simulink model "DemonstratorSimscape"  (R2020b)
settings: Solver=ode113  StartTime=0.0  StopTime=t_stop*0+20  FixedStep=1e-4
values from neighbouring files (symbols this model uses):
  brkD = 0    [main.m]
  brkI = 1e4    (= 10000)    [main.m]
  brkP = 1e5    (= 100000)    [main.m]
  d_drm = 0.5*d_drum    [main.m]
  d_shm = 0.4*d_sheave    [main.m]
  DeltaCable0 = 0    [main.m]
  Droop_scaling = 0    [main.m]
  eta_sh = 0.015    [main.m]
  filt_NUM = ones(1,200)*0.005    [main.m]
  g = 9.80665    [main.m]
  Iw = 0.5*(W.i + M.in*GB.r^2)    [main.m]
  Kp_mul = 0.3    [main.m]
  Lc0 = abs((T.ph-L.height-P.d-L.z0)*0.001)    [main.m]
  Ls1 = ((T.ph-0.5*W.pd)/1000)    [main.m]
  Ls2 = ((0.5*(T.s2+P.d)-2*P.d)/1000)    [main.m]
  M = 50e3    (= 50000)    [calcGrav.m]
  phi0_drm = -90    [main.m]
  phi0_shm = -90    [main.m]
  r_sheave = P.d*0.5    [main.m]
  s = tf('s')    [calcGrav.m]
  tau_brk = 0.001    [main.m]
  tau_em = 60e-3    (= 0.06)    [calcGrav.m]    (also in main.m)
  tau_m = tau_w/GB.r    [main.m]
  Tmax = 400e3    (= 400000)    [main.m]
  Tn_mul = 10    [main.m]
  x_drm = 0.7*r_drum    [main.m]
  x_shm = 0.7*r_sheave    [main.m]
  z0 = 0    [calcGrav.m]    (also in main.m = L.z0-P.d*0.5-P.d-P.d-L.height-T.h1-T.h2-32)
undefined symbols (not defined in the file or in its folder): C, CA, Controller_sampleTime, DiscIntNeverNeededParam, GB, L, P, Part, T, VFD_acceleration_model_factor, VFD_Adapt_factor_lower_p1458, VFD_Adapt_factor_upper_p1459, VFD_Curr_limit_var_p0641, VFD_Current_limit_p0640, VFD_Id_setp_total_r1624, VFD_Iq, VFD_Kp_n_basic_p1460, VFD_M, VFD_M_accel_T_smooth_p1517, VFD_M_lim_var_fixS_src_p1551, VFD_M_max_lower_p1521, VFD_M_max_lower_scal_p1525, VFD_M_max_up_mot_scal_p1524, VFD_M_max_upper_p1520, VFD_n_act_T_smooth_p1442, VFD_n_ctr_Kp_n_up_scal_p1461, VFD_n_ctr_Tn_n_up_sca_p1463, VFD_n_ctrl_adapt_Kp_lower_p1456, VFD_n_ctrl_adapt_Kp_upper_p1457, VFD_n_ctrl_Adpt_sig_Kp_p1455, VFD_n_ctrl_Kp_scal_p1466, VFD_n_ctrl_n_lower_p1464, VFD_n_ctrl_n_upper_p1465, VFD_n_ctrl_Tn_n_lower_p1462, VFD_n_limit_neg_p1086, VFD_n_limit_pos_p1083, VFD_n_limit_setp_p1063, VFD_n_max_p1082, VFD_n_set_filt_1_T_p1416, VFD_P_max_gen_p1531, VFD_P_max_mot_p1530, VFD_PU_I_outp_max_r0289, VFD_RFG_ramp_down_time_p1121, VFD_RFG_ramp_up_time_p1120, VFD_RFG_t_RD_scal_p1139, VFD_RFG_t_RU_scal_p1138, VSD, W, X, Y, Z
libraries: sm_lib x248, nesl_utility x128, simulink x49, pid_lib x4, cstblocks x2, simulink_extras x2
(part 6 of 10)

== system DemonstratorSimscape/Transmission System/Anchor and Load/FlexDisp_Left/L_23 ==
  L(t)[m] : Inport
  a[m/s^2] : Inport  Port=2
  Constant : Constant  Value=C.EA
  Constant1 : Constant  Value=C.dr
  Constant2 : Constant  Value=Part.m
  Constant3 : Constant  Value=g
  Constant4 : Constant  Value=C.drK
  Gain : Gain  Gain=1/Part.m
  Integrator : Integrator
  Integrator1 : Integrator
  Product : Product  Inputs=*/
  Product{1..3,5} (4 alike) : Product
  Product4 : Product  Inputs=*/
  Product6 : Product  Inputs=/*
  SW_b : ManualSwitch  CurrentSetting=0
  Sqrt : Sqrt  SaturateOnIntegerOverflow=on
  Sum1 : Sum  Inputs=+++
  Sum2 : Sum  Inputs=-+
  F[N] : Outport  VectorParamsAs1DForOutWhenUnconnected=off
  ext [m] : Outport  Port=2  VectorParamsAs1DForOutWhenUnconnected=off
  ext speed [m/s] : Outport  Port=3  VectorParamsAs1DForOutWhenUnconnected=off
  wires:
  L(t)[m]/1 -> Product/2
  Constant/1 -> Product/1
  Product2/1 -> Sum1/1
  Product3/1 -> Sum1/3
  Sum2/1 -> Product4/1, F[N]/1
  Product/1 -> Gain/1, Product2/2  "k"
  Constant2/1 -> Product4/2, Product5/2, Product3/2
  Integrator/1 -> ext speed [m/s]/1, Product1/2, Integrator1/1
  Integrator1/1 -> Product2/1, ext [m]/1
  Product4/1 -> Integrator/1
  Product1/1 -> Sum1/2
  a[m/s^2]/1 -> Product3/1
  Sum1/1 -> Sum2/1
  Product5/1 -> Sum2/2
  Constant3/1 -> Product5/1
  Gain/1 -> Sqrt/1
  Sqrt/1 -> Product6/1
  Constant4/1 -> Product6/2
  Constant1/1 -> SW_b/2
  Product6/1 -> SW_b/1
  SW_b/1 -> Product1/1

== system DemonstratorSimscape/Transmission System/Anchor and Load/FlexDisp_Left/L_34 ==
  L(t)[m] : Inport
  a[m/s^2] : Inport  Port=2
  Constant : Constant  Value=C.EA
  Constant1 : Constant  Value=C.dr
  Constant2 : Constant  Value=Part.m
  Constant3 : Constant  Value=g
  Constant4 : Constant  Value=C.drK
  Gain : Gain  Gain=1/Part.m
  Integrator : Integrator
  Integrator1 : Integrator
  Product : Product  Inputs=*/
  Product{1..3,5} (4 alike) : Product
  Product4 : Product  Inputs=*/
  Product6 : Product  Inputs=/*
  SW_b : ManualSwitch  CurrentSetting=0
  Sqrt : Sqrt  SaturateOnIntegerOverflow=on
  Sum1 : Sum  Inputs=+++
  Sum2 : Sum  Inputs=-+
  F[N] : Outport  VectorParamsAs1DForOutWhenUnconnected=off
  ext [m] : Outport  Port=2  VectorParamsAs1DForOutWhenUnconnected=off
  ext speed [m/s] : Outport  Port=3  VectorParamsAs1DForOutWhenUnconnected=off
  wires:
  L(t)[m]/1 -> Product/2
  Constant/1 -> Product/1
  Product2/1 -> Sum1/1
  Product3/1 -> Sum1/3
  Sum2/1 -> Product4/1, F[N]/1
  Product/1 -> Gain/1, Product2/2  "k"
  Constant2/1 -> Product4/2, Product5/2, Product3/2
  Integrator/1 -> ext speed [m/s]/1, Product1/2, Integrator1/1
  Integrator1/1 -> Product2/1, ext [m]/1
  Product4/1 -> Integrator/1
  Product1/1 -> Sum1/2
  a[m/s^2]/1 -> Product3/1
  Sum1/1 -> Sum2/1
  Product5/1 -> Sum2/2
  Constant3/1 -> Product5/1
  Gain/1 -> Sqrt/1
  Sqrt/1 -> Product6/1
  Constant4/1 -> Product6/2
  Constant1/1 -> SW_b/2
  Product6/1 -> SW_b/1
  SW_b/1 -> Product1/1

== system DemonstratorSimscape/Transmission System/Anchor and Load/FlexDisp_Left/L_w1 ==
  L(t)[m] : Inport
  a[m/s^2] : Inport  Port=2
  Constant : Constant  Value=C.EA
  Constant1 : Constant  Value=C.dr
  Constant2 : Constant  Value=Part.m
  Constant3 : Constant  Value=g
  Constant4 : Constant  Value=C.drK
  Gain : Gain  Gain=1/Part.m
  Integrator : Integrator
  Integrator1 : Integrator
  Product : Product  Inputs=*/
  Product{1..3,5} (4 alike) : Product
  Product4 : Product  Inputs=*/
  Product6 : Product  Inputs=/*
  SW_b : ManualSwitch  CurrentSetting=0
  Sqrt : Sqrt  SaturateOnIntegerOverflow=on
  Sum1 : Sum  Inputs=+++
  Sum2 : Sum  Inputs=-+
  F[N] : Outport  VectorParamsAs1DForOutWhenUnconnected=off
  ext [m] : Outport  Port=2  VectorParamsAs1DForOutWhenUnconnected=off
  ext speed [m/s] : Outport  Port=3  VectorParamsAs1DForOutWhenUnconnected=off
  wires:
  L(t)[m]/1 -> Product/2
  Constant/1 -> Product/1
  Product2/1 -> Sum1/1
  Product3/1 -> Sum1/3
  Sum2/1 -> Product4/1, F[N]/1
  Product/1 -> Gain/1, Product2/2  "k"
  Constant2/1 -> Product4/2, Product5/2, Product3/2
  Integrator/1 -> ext speed [m/s]/1, Product1/2, Integrator1/1
  Integrator1/1 -> Product2/1, ext [m]/1
  Product4/1 -> Integrator/1
  Product1/1 -> Sum1/2
  a[m/s^2]/1 -> Product3/1
  Sum1/1 -> Sum2/1
  Product5/1 -> Sum2/2
  Constant3/1 -> Product5/1
  Gain/1 -> Sqrt/1
  Sqrt/1 -> Product6/1
  Constant4/1 -> Product6/2
  Constant1/1 -> SW_b/2
  Product6/1 -> SW_b/1
  SW_b/1 -> Product1/1

== system DemonstratorSimscape/Transmission System/Anchor and Load/FlexDisp_Right/L_54 ==
  L(t)[m] : Inport
  a[m/s^2] : Inport  Port=2
  Constant : Constant  Value=C.EA
  Constant1 : Constant  Value=C.dr
  Constant2 : Constant  Value=Part.m
  Constant3 : Constant  Value=g
  Constant4 : Constant  Value=C.drK
  Gain : Gain  Gain=1/Part.m
  Integrator : Integrator
  Integrator1 : Integrator
  Product : Product  Inputs=*/
  Product{1..3,5} (4 alike) : Product
  Product4 : Product  Inputs=*/
  Product6 : Product  Inputs=/*
  SW_b : ManualSwitch  CurrentSetting=0
  Sqrt : Sqrt  SaturateOnIntegerOverflow=on
  Sum1 : Sum  Inputs=+++
  Sum2 : Sum  Inputs=-+
  F[N] : Outport  VectorParamsAs1DForOutWhenUnconnected=off
  ext [m] : Outport  Port=2  VectorParamsAs1DForOutWhenUnconnected=off
  ext speed [m/s] : Outport  Port=3  VectorParamsAs1DForOutWhenUnconnected=off
  wires:
  L(t)[m]/1 -> Product/2
  Constant/1 -> Product/1
  Product2/1 -> Sum1/1
  Product3/1 -> Sum1/3
  Sum2/1 -> Product4/1, F[N]/1
  Product/1 -> Gain/1, Product2/2  "k"
  Constant2/1 -> Product4/2, Product5/2, Product3/2
  Integrator/1 -> ext speed [m/s]/1, Product1/2, Integrator1/1
  Integrator1/1 -> Product2/1, ext [m]/1
  Product4/1 -> Integrator/1
  Product1/1 -> Sum1/2
  a[m/s^2]/1 -> Product3/1
  Sum1/1 -> Sum2/1
  Product5/1 -> Sum2/2
  Constant3/1 -> Product5/1
  Gain/1 -> Sqrt/1
  Sqrt/1 -> Product6/1
  Constant4/1 -> Product6/2
  Constant1/1 -> SW_b/2
  Product6/1 -> SW_b/1
  SW_b/1 -> Product1/1

== system DemonstratorSimscape/Transmission System/Anchor and Load/FlexDisp_Right/L_65 ==
  L(t)[m] : Inport
  a[m/s^2] : Inport  Port=2
  Constant : Constant  Value=C.EA
  Constant1 : Constant  Value=C.dr
  Constant2 : Constant  Value=Part.m
  Constant3 : Constant  Value=g
  Constant4 : Constant  Value=C.drK
  Gain : Gain  Gain=1/Part.m
  Integrator : Integrator
  Integrator1 : Integrator
  Product : Product  Inputs=*/
  Product{1..3,5} (4 alike) : Product
  Product4 : Product  Inputs=*/
  Product6 : Product  Inputs=/*
  SW_b : ManualSwitch  CurrentSetting=0
  Sqrt : Sqrt  SaturateOnIntegerOverflow=on
  Sum1 : Sum  Inputs=+++
  Sum2 : Sum  Inputs=-+
  F[N] : Outport  VectorParamsAs1DForOutWhenUnconnected=off
  ext [m] : Outport  Port=2  VectorParamsAs1DForOutWhenUnconnected=off
  ext speed [m/s] : Outport  Port=3  VectorParamsAs1DForOutWhenUnconnected=off
  wires:
  L(t)[m]/1 -> Product/2
  Constant/1 -> Product/1
  Product2/1 -> Sum1/1
  Product3/1 -> Sum1/3
  Sum2/1 -> Product4/1, F[N]/1
  Product/1 -> Gain/1, Product2/2  "k"
  Constant2/1 -> Product4/2, Product5/2, Product3/2
  Integrator/1 -> ext speed [m/s]/1, Product1/2, Integrator1/1
  Integrator1/1 -> Product2/1, ext [m]/1
  Product4/1 -> Integrator/1
  Product1/1 -> Sum1/2
  a[m/s^2]/1 -> Product3/1
  Sum1/1 -> Sum2/1
  Product5/1 -> Sum2/2
  Constant3/1 -> Product5/1
  Gain/1 -> Sqrt/1
  Sqrt/1 -> Product6/1
  Constant4/1 -> Product6/2
  Constant1/1 -> SW_b/2
  Product6/1 -> SW_b/1
  SW_b/1 -> Product1/1

== system DemonstratorSimscape/Transmission System/Anchor and Load/FlexDisp_Right/L_76 ==
  L(t)[m] : Inport
  a[m/s^2] : Inport  Port=2
  Constant : Constant  Value=C.EA
  Constant1 : Constant  Value=C.dr
  Constant2 : Constant  Value=Part.m
  Constant3 : Constant  Value=g
  Constant4 : Constant  Value=C.drK
  Gain : Gain  Gain=1/Part.m
  Integrator : Integrator
  Integrator1 : Integrator
  Product : Product  Inputs=*/
  Product{1..3,5} (4 alike) : Product
  Product4 : Product  Inputs=*/
  Product6 : Product  Inputs=/*
  SW_b : ManualSwitch  CurrentSetting=0
  Sqrt : Sqrt  SaturateOnIntegerOverflow=on
  Sum1 : Sum  Inputs=+++
  Sum2 : Sum  Inputs=-+
  F[N] : Outport  VectorParamsAs1DForOutWhenUnconnected=off
  ext [m] : Outport  Port=2  VectorParamsAs1DForOutWhenUnconnected=off
  ext speed [m/s] : Outport  Port=3  VectorParamsAs1DForOutWhenUnconnected=off
  wires:
  L(t)[m]/1 -> Product/2
  Constant/1 -> Product/1
  Product2/1 -> Sum1/1
  Product3/1 -> Sum1/3
  Sum2/1 -> Product4/1, F[N]/1
  Product/1 -> Gain/1, Product2/2  "k"
  Constant2/1 -> Product4/2, Product5/2, Product3/2
  Integrator/1 -> ext speed [m/s]/1, Product1/2, Integrator1/1
  Integrator1/1 -> Product2/1, ext [m]/1
  Product4/1 -> Integrator/1
  Product1/1 -> Sum1/2
  a[m/s^2]/1 -> Product3/1
  Sum1/1 -> Sum2/1
  Product5/1 -> Sum2/2
  Constant3/1 -> Product5/1
  Gain/1 -> Sqrt/1
  Sqrt/1 -> Product6/1
  Constant4/1 -> Product6/2
  Constant1/1 -> SW_b/2
  Product6/1 -> SW_b/1
  SW_b/1 -> Product1/1

== system DemonstratorSimscape/Transmission System/Anchor and Load/FlexDisp_Right/L_w7 ==
  L(t)[m] : Inport
  a[m/s^2] : Inport  Port=2
  Constant : Constant  Value=C.EA
  Constant1 : Constant  Value=C.dr
  Constant2 : Constant  Value=Part.m
  Constant3 : Constant  Value=g
  Constant4 : Constant  Value=C.drK
  Gain : Gain  Gain=1/Part.m
  Integrator : Integrator
  Integrator1 : Integrator
  Product : Product  Inputs=*/
  Product{1..3,5} (4 alike) : Product
  Product4 : Product  Inputs=*/
  Product6 : Product  Inputs=/*
  SW_b : ManualSwitch  CurrentSetting=0
  Sqrt : Sqrt  SaturateOnIntegerOverflow=on
  Sum1 : Sum  Inputs=+++
  Sum2 : Sum  Inputs=-+
  F[N] : Outport  VectorParamsAs1DForOutWhenUnconnected=off
  ext [m] : Outport  Port=2  VectorParamsAs1DForOutWhenUnconnected=off
  ext speed [m/s] : Outport  Port=3  VectorParamsAs1DForOutWhenUnconnected=off
  wires:
  L(t)[m]/1 -> Product/2
  Constant/1 -> Product/1
  Product2/1 -> Sum1/1
  Product3/1 -> Sum1/3
  Sum2/1 -> Product4/1, F[N]/1
  Product/1 -> Gain/1, Product2/2  "k"
  Constant2/1 -> Product4/2, Product5/2, Product3/2
  Integrator/1 -> ext speed [m/s]/1, Product1/2, Integrator1/1
  Integrator1/1 -> Product2/1, ext [m]/1
  Product4/1 -> Integrator/1
  Product1/1 -> Sum1/2
  a[m/s^2]/1 -> Product3/1
  Sum1/1 -> Sum2/1
  Product5/1 -> Sum2/2
  Constant3/1 -> Product5/1
  Gain/1 -> Sqrt/1
  Sqrt/1 -> Product6/1
  Constant4/1 -> Product6/2
  Constant1/1 -> SW_b/2
  Product6/1 -> SW_b/1
  SW_b/1 -> Product1/1

== system DemonstratorSimscape/Transmission System/Anchor and Load/Load/DOUBLE ==
  cable mass : Inport
  " 1" : sm_lib/Frames and Transforms/Rigid Transform  TranslationMethod=Cartesian  TranslationStandardOffset=0  TranslationLengthUnit=mm  TranslationStandardAxis=+Z  TranslationCartesianOffset=[0 -P.d*0.5 0 ]  TranslationROffset=0  TranslationROffsetUnits=m  TranslationZOffset=0  TranslationZOffsetUnits=m  TranslationThetaOffset=0  TranslationThetaOffsetUnits=deg  RotationMethod=None  RotationAngleUnits=deg  RotationStandardAxis=+Z  RotationAngle=0  RotationArbitraryAxis=[0 0 1]  FollAlignAxisA=+X  BaseAlignAxisA=+Y  FollAlignAxisB=+Y  BaseAlignAxisB=+Z  RotationSequenceAxes=FollowerAxes  RotationSequence=XYX  RotationSequenceAngles=[0 0 0]  RotationSequenceAnglesUnits=deg  RotationMatrix=[1 0 0; 0 1 0; 0 0 1]
  " 2" : sm_lib/Frames and Transforms/Rigid Transform  TranslationMethod=Cartesian  TranslationStandardOffset=0  TranslationLengthUnit=mm  TranslationStandardAxis=+Z  TranslationCartesianOffset=[0 -P.d*0.5 0 ]  TranslationROffset=0  TranslationROffsetUnits=m  TranslationZOffset=0  TranslationZOffsetUnits=m  TranslationThetaOffset=0  TranslationThetaOffsetUnits=deg  RotationMethod=None  RotationAngleUnits=deg  RotationStandardAxis=+Z  RotationAngle=0  RotationArbitraryAxis=[0 0 1]  FollAlignAxisA=+X  BaseAlignAxisA=+Y  FollAlignAxisB=+Y  BaseAlignAxisB=+Z  RotationSequenceAxes=FollowerAxes  RotationSequence=XYX  RotationSequenceAngles=[0 0 0]  RotationSequenceAnglesUnits=deg  RotationMatrix=[1 0 0; 0 1 0; 0 0 1]
  Cable_Left : Subsystem
  Cable_Right : Subsystem
  Half-Place R : sm_lib/Body Elements/Brick Solid  GraphicAmbientColor=[0.15 0.15 0.15 1.0]  BasedOnType=Mass  BrickDimensions=[L.ap*2 P.d 1.5*P.h]  BrickDimensionUnits=mm  CenterOfMass=[0 0 0]  CenterOfMassUnits=m  GraphicDiffuseColor=c.plate  Density=0  DensityUnits=g/cm^3  DoExposeReferenceFrame=on  GraphicEmissiveColor=[0.0 0.0 0.0 1.0]  ExportEntireGeometry=off  SerializedFrames=<Frames/>  MarkerShape=Sphere  MarkerSize=10  GraphicType=FromGeometry  InertiaType=CalculateFromGeometry  Mass=L.cpmass/2  MassUnits=kg  MomentsOfInertia=[1 1 1]  MomentsOfInertiaUnits=kg*m^2  GraphicOpacity=c.opac  ProductsOfInertia=[0 0 0]  ProductsOfInertiaUnits=kg*m^2  GraphicShininess=75  GraphicSpecularColor=[0.5 0.5 0.5 1.0]  GraphicVisPropType=SimpleVisualProperties
  Half-Plate L : sm_lib/Body Elements/Brick Solid  GraphicAmbientColor=[0.15 0.15 0.15 1.0]  BasedOnType=Mass  BrickDimensions=[L.ap*2 P.d 1.5*P.h]  BrickDimensionUnits=mm  CenterOfMass=[0 0 0]  CenterOfMassUnits=m  GraphicDiffuseColor=c.plate  Density=0  DensityUnits=g/cm^3  DoExposeReferenceFrame=on  GraphicEmissiveColor=[0.0 0.0 0.0 1.0]  ExportEntireGeometry=off  SerializedFrames=<Frames/>  MarkerShape=Sphere  MarkerSize=10  GraphicType=FromGeometry  InertiaType=CalculateFromGeometry  Mass=L.cpmass/2  MassUnits=kg  MomentsOfInertia=[1 1 1]  MomentsOfInertiaUnits=kg*m^2  GraphicOpacity=c.opac  ProductsOfInertia=[0 0 0]  ProductsOfInertiaUnits=kg*m^2  GraphicShininess=75  GraphicSpecularColor=[0.5 0.5 0.5 1.0]  GraphicVisPropType=SimpleVisualProperties
  Load blue : sm_lib/Body Elements/Brick Solid  GraphicAmbientColor=[0.15 0.15 0.15 1.0]  BasedOnType=Mass  BrickDimensions="[L.width L.height  L.depth]"  BrickDimensionUnits=mm  CenterOfMass=[0 0 0]  CenterOfMassUnits=m  GraphicDiffuseColor=c.Rload  Density=L.den  DensityUnits=g/cm^3  DoExposeReferenceFrame=off  GraphicEmissiveColor=[0.0 0.0 0.0 1.0]  ExportEntireGeometry=off  SerializedFrames=<Frames><Frame><Id>Frame1</Id><Value><Name>F</Name><Origin><Source>ReferenceFrame</Source><FeatureName></FeatureName></Origin><PrimaryAxis><DefinedDirection>+Z</DefinedDirection><Source>ReferenceFrame</Source><SourceDirection>+Z</SourceDirection><FeatureName></FeatureName></PrimaryAxis><SecondaryAxis><DefinedDirection>+X</DefinedDirection><Source>ReferenceFrame</Source><SourceDirection>+X</SourceDirection><FeatureName></FeatureName></SecondaryAxis></Value></Frame></Frames>  MarkerShape=Sphere  MarkerSize=10  GraphicType=FromGeometry  InertiaType=CalculateFromGeometry  Mass=L.mass  MassUnits=kg  MomentsOfInertia=[0 0 0]  MomentsOfInertiaUnits=kg*m^2  GraphicOpacity=1.0  ProductsOfInertia=[0 0 0]  ProductsOfInertiaUnits=kg*m^2  GraphicShininess=75  GraphicSpecularColor=[0.5 0.5 0.5 1.0]  GraphicVisPropType=SimpleVisualProperties
  Load init position1 : sm_lib/Frames and Transforms/Rigid Transform  TranslationMethod=Cartesian  TranslationStandardOffset=0  TranslationLengthUnit=mm  TranslationStandardAxis=+Z  TranslationCartesianOffset=[0 -P.d*0.5-L.height*0.5 -P.h*.5 ]  TranslationROffset=0  TranslationROffsetUnits=m  TranslationZOffset=0  TranslationZOffsetUnits=m  TranslationThetaOffset=0  TranslationThetaOffsetUnits=deg  RotationMethod=StandardAxis  RotationAngleUnits=deg  RotationStandardAxis=+Y  RotationAngle=180  RotationArbitraryAxis=[0 0 1]  FollAlignAxisA=+X  BaseAlignAxisA=+Y  FollAlignAxisB=+Y  BaseAlignAxisB=+Z  RotationSequenceAxes=FollowerAxes  RotationSequence=XYX  RotationSequenceAngles=[0 0 0]  RotationSequenceAnglesUnits=deg  RotationMatrix=[1 0 0; 0 1 0; 0 0 1]
  Load init position2 : sm_lib/Frames and Transforms/Rigid Transform  TranslationMethod=Cartesian  TranslationStandardOffset=0  TranslationLengthUnit=mm  TranslationStandardAxis=+Z  TranslationCartesianOffset=[0 -L.height*.5-P.d 0 ]  TranslationROffset=0  TranslationROffsetUnits=m  TranslationZOffset=0  TranslationZOffsetUnits=m  TranslationThetaOffset=0  TranslationThetaOffsetUnits=deg  RotationMethod=None  RotationAngleUnits=deg  RotationStandardAxis=+X  RotationAngle=180  RotationArbitraryAxis=[0 0 1]  FollAlignAxisA=+X  BaseAlignAxisA=+Y  FollAlignAxisB=+Y  BaseAlignAxisB=+Z  RotationSequenceAxes=FollowerAxes  RotationSequence=XYX  RotationSequenceAngles=[0 0 0]  RotationSequenceAnglesUnits=deg  RotationMatrix=[1 0 0; 0 1 0; 0 0 1]
  Load init position3 : sm_lib/Frames and Transforms/Rigid Transform  TranslationMethod=Cartesian  TranslationStandardOffset=0  TranslationLengthUnit=mm  TranslationStandardAxis=+Z  TranslationCartesianOffset=[0 -L.height*.5-P.d 0 ]  TranslationROffset=0  TranslationROffsetUnits=m  TranslationZOffset=0  TranslationZOffsetUnits=m  TranslationThetaOffset=0  TranslationThetaOffsetUnits=deg  RotationMethod=None  RotationAngleUnits=deg  RotationStandardAxis=+X  RotationAngle=180  RotationArbitraryAxis=[0 0 1]  FollAlignAxisA=+X  BaseAlignAxisA=+Y  FollAlignAxisB=+Y  BaseAlignAxisB=+Z  RotationSequenceAxes=FollowerAxes  RotationSequence=XYX  RotationSequenceAngles=[0 0 0]  RotationSequenceAnglesUnits=deg  RotationMatrix=[1 0 0; 0 1 0; 0 0 1]
  Load init position4 : sm_lib/Frames and Transforms/Rigid Transform  TranslationMethod=Cartesian  TranslationStandardOffset=0  TranslationLengthUnit=mm  TranslationStandardAxis=+Z  TranslationCartesianOffset=[0 -P.d*0.5-L.height*0.5 -P.h*.5 ]  TranslationROffset=0  TranslationROffsetUnits=m  TranslationZOffset=0  TranslationZOffsetUnits=m  TranslationThetaOffset=0  TranslationThetaOffsetUnits=deg  RotationMethod=StandardAxis  RotationAngleUnits=deg  RotationStandardAxis=+Y  RotationAngle=180  RotationArbitraryAxis=[0 0 1]  FollAlignAxisA=+X  BaseAlignAxisA=+Y  FollAlignAxisB=+Y  BaseAlignAxisB=+Z  RotationSequenceAxes=FollowerAxes  RotationSequence=XYX  RotationSequenceAngles=[0 0 0]  RotationSequenceAnglesUnits=deg  RotationMatrix=[1 0 0; 0 1 0; 0 0 1]
  Load yellow : sm_lib/Body Elements/Brick Solid  GraphicAmbientColor=[0.15 0.15 0.15 1.0]  BasedOnType=Mass  BrickDimensions="[L.width L.height  L.depth]"  BrickDimensionUnits=mm  CenterOfMass=[0 0 0]  CenterOfMassUnits=m  GraphicDiffuseColor=[1.0 1.0 0.0]  Density=L.den  DensityUnits=g/cm^3  DoExposeReferenceFrame=off  GraphicEmissiveColor=[0.0 0.0 0.0 1.0]  ExportEntireGeometry=off  SerializedFrames=<Frames><Frame><Id>Frame1</Id><Value><Name>F</Name><Origin><Source>ReferenceFrame</Source><FeatureName></FeatureName></Origin><PrimaryAxis><DefinedDirection>+Z</DefinedDirection><Source>ReferenceFrame</Source><SourceDirection>+Z</SourceDirection><FeatureName></FeatureName></PrimaryAxis><SecondaryAxis><DefinedDirection>+X</DefinedDirection><Source>ReferenceFrame</Source><SourceDirection>+X</SourceDirection><FeatureName></FeatureName></SecondaryAxis></Value></Frame></Frames>  MarkerShape=Sphere  MarkerSize=10  GraphicType=FromGeometry  InertiaType=CalculateFromGeometry  Mass=L.mass  MassUnits=kg  MomentsOfInertia=[0 0 0]  MomentsOfInertiaUnits=kg*m^2  GraphicOpacity=1.0  ProductsOfInertia=[0 0 0]  ProductsOfInertiaUnits=kg*m^2  GraphicShininess=75  GraphicSpecularColor=[0.5 0.5 0.5 1.0]  GraphicVisPropType=SimpleVisualProperties
  Load1 Rotation1 : sm_lib/Frames and Transforms/Rigid Transform  TranslationMethod=None  TranslationStandardOffset=0  TranslationLengthUnit=m  TranslationStandardAxis=+Z  TranslationCartesianOffset=[0 0 0]  TranslationROffset=0  TranslationROffsetUnits=m  TranslationZOffset=0  TranslationZOffsetUnits=m  TranslationThetaOffset=0  TranslationThetaOffsetUnits=deg  RotationMethod=StandardAxis  RotationAngleUnits=deg  RotationStandardAxis=+X  RotationAngle=90  RotationArbitraryAxis=[0 0 1]  FollAlignAxisA=+Y  BaseAlignAxisA=-Z  FollAlignAxisB=+X  BaseAlignAxisB=+X  RotationSequenceAxes=FollowerAxes  RotationSequence=XYX  RotationSequenceAngles=[0 0 0]  RotationSequenceAnglesUnits=deg  RotationMatrix=[1 0 0; 0 1 0; 0 0 1]
  Load1 Rotation2 : sm_lib/Frames and Transforms/Rigid Transform  TranslationMethod=None  TranslationStandardOffset=0  TranslationLengthUnit=m  TranslationStandardAxis=+Z  TranslationCartesianOffset=[0 0 0]  TranslationROffset=0  TranslationROffsetUnits=m  TranslationZOffset=0  TranslationZOffsetUnits=m  TranslationThetaOffset=0  TranslationThetaOffsetUnits=deg  RotationMethod=StandardAxis  RotationAngleUnits=deg  RotationStandardAxis=+X  RotationAngle=90  RotationArbitraryAxis=[0 0 1]  FollAlignAxisA=+Y  BaseAlignAxisA=-Z  FollAlignAxisB=+X  BaseAlignAxisB=+X  RotationSequenceAxes=FollowerAxes  RotationSequence=XYX  RotationSequenceAngles=[0 0 0]  RotationSequenceAnglesUnits=deg  RotationMatrix=[1 0 0; 0 1 0; 0 0 1]
  Planar Load1 : Subsystem
  Planar Load2 : Subsystem
  Rigid Transform1 : sm_lib/Frames and Transforms/Rigid Transform  TranslationMethod=Cartesian  TranslationStandardOffset=0  TranslationLengthUnit=mm  TranslationStandardAxis=+Z  TranslationCartesianOffset=[0 0.5*T.rs 0]  TranslationROffset=0  TranslationROffsetUnits=m  TranslationZOffset=0  TranslationZOffsetUnits=m  TranslationThetaOffset=0  TranslationThetaOffsetUnits=deg  RotationMethod=StandardAxis  RotationAngleUnits=deg  RotationStandardAxis=+Y  RotationAngle=180  RotationArbitraryAxis=[1 0 0]  FollAlignAxisA=+X  BaseAlignAxisA=+Y  FollAlignAxisB=+Y  BaseAlignAxisB=+Z  RotationSequenceAxes=FollowerAxes  RotationSequence=XYX  RotationSequenceAngles=[0 0 0]  RotationSequenceAnglesUnits=deg  RotationMatrix=[1 0 0; 0 1 0; 0 0 1]
  Rigid Transform2 : sm_lib/Frames and Transforms/Rigid Transform  TranslationMethod=Cartesian  TranslationStandardOffset=0  TranslationLengthUnit=mm  TranslationStandardAxis=+Z  TranslationCartesianOffset=[0 0.5*T.rs 0]  TranslationROffset=0  TranslationROffsetUnits=m  TranslationZOffset=0  TranslationZOffsetUnits=m  TranslationThetaOffset=0  TranslationThetaOffsetUnits=deg  RotationMethod=StandardAxis  RotationAngleUnits=deg  RotationStandardAxis=+Y  RotationAngle=180  RotationArbitraryAxis=[1 0 0]  FollAlignAxisA=+X  BaseAlignAxisA=+Y  FollAlignAxisB=+Y  BaseAlignAxisB=+Z  RotationSequenceAxes=FollowerAxes  RotationSequence=XYX  RotationSequenceAngles=[0 0 0]  RotationSequenceAnglesUnits=deg  RotationMatrix=[1 0 0; 0 1 0; 0 0 1]
  Rigid Transform3 : sm_lib/Frames and Transforms/Rigid Transform  TranslationMethod=Cartesian  TranslationStandardOffset=0  TranslationLengthUnit=mm  TranslationStandardAxis=+Z  TranslationCartesianOffset=[-0.5*(P.Bd+P.d) 0 0]  TranslationROffset=0  TranslationROffsetUnits=m  TranslationZOffset=0  TranslationZOffsetUnits=m  TranslationThetaOffset=0  TranslationThetaOffsetUnits=deg  RotationMethod=StandardAxis  RotationAngleUnits=deg  RotationStandardAxis=+Z  RotationAngle=180  RotationArbitraryAxis=[1 0 0]  FollAlignAxisA=+X  BaseAlignAxisA=+Y  FollAlignAxisB=+Y  BaseAlignAxisB=+Z  RotationSequenceAxes=FollowerAxes  RotationSequence=XYX  RotationSequenceAngles=[0 0 0]  RotationSequenceAnglesUnits=deg  RotationMatrix=[1 0 0; 0 1 0; 0 0 1]
  Rigid Transform4 : sm_lib/Frames and Transforms/Rigid Transform  TranslationMethod=Cartesian  TranslationStandardOffset=0  TranslationLengthUnit=mm  TranslationStandardAxis=+Z  TranslationCartesianOffset=[0.5*(P.Bd+P.d) 0 0]  TranslationROffset=0  TranslationROffsetUnits=m  TranslationZOffset=0  TranslationZOffsetUnits=m  TranslationThetaOffset=0  TranslationThetaOffsetUnits=deg  RotationMethod=StandardAxis  RotationAngleUnits=deg  RotationStandardAxis=+Z  RotationAngle=180  RotationArbitraryAxis=[1 0 0]  FollAlignAxisA=+X  BaseAlignAxisA=+Y  FollAlignAxisB=+Y  BaseAlignAxisB=+Z  RotationSequenceAxes=FollowerAxes  RotationSequence=XYX  RotationSequenceAngles=[0 0 0]  RotationSequenceAnglesUnits=deg  RotationMatrix=[1 0 0; 0 1 0; 0 0 1]
  Conn1 : PMIOPort  Side=Left
  Pulley low 1 : PMIOPort  Port=2  Side=Right
  Pullley low 2 : PMIOPort  Port=3  Side=Right
  LoadFrame : PMIOPort  Port=4  Side=Left
  wires:
  cable mass/1 -> Cable_Right/1(In1), Cable_Left/1(In1)
  connections:
  Load1 Rotation1/LConn1 -- Planar Load1/RConn1
  Load init position2/LConn1 -- Load1 Rotation1/RConn1
  Planar Load1/LConn1 -- Rigid Transform3/RConn1
  Pulley low 1/RConn1 -- Load init position2/RConn1 -- Rigid Transform2/RConn1
  Pullley low 2/RConn1 -- Load init position3/RConn1 -- Rigid Transform1/RConn1
  " 1"/LConn1 -- Rigid Transform2/LConn1 -- Cable_Left/RConn1
  " 2"/LConn1 -- Rigid Transform1/LConn1 -- Cable_Right/RConn1
  Half-Plate L/RConn1 -- " 1"/RConn1 -- Load init position1/LConn1
  Half-Place R/RConn1 -- " 2"/RConn1 -- Load init position4/LConn1
  Load yellow/LConn1 -- Load init position1/RConn1
  Load blue/LConn1 -- LoadFrame/RConn1 -- Load init position4/RConn1
  Load1 Rotation2/LConn1 -- Planar Load2/RConn1
  Load1 Rotation2/RConn1 -- Load init position3/LConn1
  Conn1/RConn1 -- Rigid Transform4/LConn1 -- Rigid Transform3/LConn1
  Planar Load2/LConn1 -- Rigid Transform4/RConn1

== system DemonstratorSimscape/Transmission System/Anchor and Load/Load/Load Sensors ==
  Constant : Constant  Value=L.height*0.5
  Load : Scope  NumInputPorts=3
  PS-Simulink Converter : nesl_utility/PS-Simulink Converter  PhysicalDomain=network_engine_domain  SubClassName=ps_output  LeftPortType=input  RightPortType=output  PseudoPeriodic=off  Frequencies=[]  Unit=mm  AffineConversion=off
  PS-Simulink Converter1 : nesl_utility/PS-Simulink Converter  PhysicalDomain=network_engine_domain  SubClassName=ps_output  LeftPortType=input  RightPortType=output  PseudoPeriodic=off  Frequencies=[]  Unit=m/s  AffineConversion=off
  PS-Simulink Converter2 : nesl_utility/PS-Simulink Converter  PhysicalDomain=network_engine_domain  SubClassName=ps_output  LeftPortType=input  RightPortType=output  PseudoPeriodic=off  Frequencies=[]  Unit=m/s^2  AffineConversion=off
  Sum : Sum  Inputs=-+
  Transform Sensor : sm_lib/Frames and Transforms/Transform Sensor  MeasurementFrame=World  SenseAngle=off  SenseAxis=off  SenseAngle1=off  SenseAngle2=off  SenseAngle3=off  SenseQ=on  SenseR=off  SenseOmegaX=off  SenseOmegaY=off  SenseOmegaZ=off  SenseOmega1=off  SenseOmega2=off  SenseOmega3=off  SenseQDot=off  SenseRDot=off  SenseAlphaX=off  SenseAlphaY=off  SenseAlphaZ=off  SenseAlpha1=off  SenseAlpha2=off  SenseAlpha3=off  SenseQDDot=off  SenseRDDot=off  SenseX=on  SenseY=on  SenseZ=off  SenseRad=off  SenseAzim=off  SenseDist=off  SenseInc=off  SenseXDot=on  SenseYDot=on  SenseZDot=off  SenseRadDot=off  SenseAzimDot=off  SenseDistDot=off  SenseIncDot=off  SenseXDDot=off  SenseYDDot=on  SenseZDDot=off  SenseRadDDot=off  SenseAzimDDot=off  SenseDistDDot=off  SenseIncDDot=off
  World Frame : sm_lib/Frames and Transforms/World Frame
  "[mm] to [m]" : Gain  Gain=0.001
  LoadFrame : PMIOPort  Side=Right
  LoadAcc (m/s^2) : Outport
  LoadPos (mm) : Outport  Port=2
  LoadVel (m/s) : Outport  Port=3
  tag scope: LoadAcc=global
  wires:
  Sum/1 -> LoadPos (mm)/1, "[mm] to [m]"/1
  Constant/1 -> Sum/1
  "[mm] to [m]"/1 -> Load/1
  PS-Simulink Converter/1 -> Sum/2
  PS-Simulink Converter2/1 -> [LoadAcc], LoadAcc (m/s^2)/1, Load/3
  PS-Simulink Converter1/1 -> LoadVel (m/s)/1, Load/2
  connections:
  Transform Sensor/RConn7 -- PS-Simulink Converter2/LConn1
  Transform Sensor/RConn4 -- PS-Simulink Converter/LConn1
  Transform Sensor/RConn6 -- PS-Simulink Converter1/LConn1
  LoadFrame/RConn1 -- Transform Sensor/RConn1
  World Frame/RConn1 -- Transform Sensor/LConn1

== system DemonstratorSimscape/Transmission System/Anchor and Load/Load/SINGLE ==
  note: Anchor
  note: Single Load
  cable mass : Inport
  " " : sm_lib/Frames and Transforms/Rigid Transform  TranslationMethod=Cartesian  TranslationStandardOffset=0  TranslationLengthUnit=mm  TranslationStandardAxis=+Z  TranslationCartesianOffset=[0 -P.d*.25 -P.h]  TranslationROffset=0  TranslationROffsetUnits=m  TranslationZOffset=0  TranslationZOffsetUnits=m  TranslationThetaOffset=0  TranslationThetaOffsetUnits=deg  RotationMethod=ArbitraryAxis  RotationAngleUnits=deg  RotationStandardAxis=+Z  RotationAngle=90  RotationArbitraryAxis=[1 0 0]  FollAlignAxisA=+X  BaseAlignAxisA=+Y  FollAlignAxisB=+Y  BaseAlignAxisB=+Z  RotationSequenceAxes=FollowerAxes  RotationSequence=XYX  RotationSequenceAngles=[0 0 0]  RotationSequenceAnglesUnits=deg  RotationMatrix=[1 0 0; 0 1 0; 0 0 1]
  " 17" : sm_lib/Frames and Transforms/Rigid Transform  TranslationMethod=Cartesian  TranslationStandardOffset=0  TranslationLengthUnit=mm  TranslationStandardAxis=+Z  TranslationCartesianOffset=[0 -P.d*0.5 0 ]  TranslationROffset=0  TranslationROffsetUnits=m  TranslationZOffset=0  TranslationZOffsetUnits=m  TranslationThetaOffset=0  TranslationThetaOffsetUnits=deg  RotationMethod=None  RotationAngleUnits=deg  RotationStandardAxis=+Z  RotationAngle=0  RotationArbitraryAxis=[0 0 1]  FollAlignAxisA=+X  BaseAlignAxisA=+Y  FollAlignAxisB=+Y  BaseAlignAxisB=+Z  RotationSequenceAxes=FollowerAxes  RotationSequence=XYX  RotationSequenceAngles=[0 0 0]  RotationSequenceAnglesUnits=deg  RotationMatrix=[1 0 0; 0 1 0; 0 0 1]
  " 3" : sm_lib/Frames and Transforms/Rigid Transform  TranslationMethod=Cartesian  TranslationStandardOffset=0  TranslationLengthUnit=mm  TranslationStandardAxis=+Z  TranslationCartesianOffset=[0 0 -T.rs ]  TranslationROffset=0  TranslationROffsetUnits=m  TranslationZOffset=0  TranslationZOffsetUnits=m  TranslationThetaOffset=0  TranslationThetaOffsetUnits=deg  RotationMethod=None  RotationAngleUnits=deg  RotationStandardAxis=+Z  RotationAngle=90  RotationArbitraryAxis=[1 0 0]  FollAlignAxisA=+X  BaseAlignAxisA=+Y  FollAlignAxisB=+Y  BaseAlignAxisB=+Z  RotationSequenceAxes=FollowerAxes  RotationSequence=XYX  RotationSequenceAngles=[0 0 0]  RotationSequenceAnglesUnits=deg  RotationMatrix=[1 0 0; 0 1 0; 0 0 1]
  " 4" : sm_lib/Frames and Transforms/Rigid Transform  TranslationMethod=Cartesian  TranslationStandardOffset=0  TranslationLengthUnit=mm  TranslationStandardAxis=+Z  TranslationCartesianOffset=[0 -P.d*.25 P.h]  TranslationROffset=0  TranslationROffsetUnits=m  TranslationZOffset=0  TranslationZOffsetUnits=m  TranslationThetaOffset=0  TranslationThetaOffsetUnits=deg  RotationMethod=ArbitraryAxis  RotationAngleUnits=deg  RotationStandardAxis=+Z  RotationAngle=90  RotationArbitraryAxis=[1 0 0]  FollAlignAxisA=+X  BaseAlignAxisA=+Y  FollAlignAxisB=+Y  BaseAlignAxisB=+Z  RotationSequenceAxes=FollowerAxes  RotationSequence=XYX  RotationSequenceAngles=[0 0 0]  RotationSequenceAnglesUnits=deg  RotationMatrix=[1 0 0; 0 1 0; 0 0 1]
  " 5" : sm_lib/Frames and Transforms/Rigid Transform  TranslationMethod=Cartesian  TranslationStandardOffset=0  TranslationLengthUnit=mm  TranslationStandardAxis=+Z  TranslationCartesianOffset=[0 0 T.rs ]  TranslationROffset=0  TranslationROffsetUnits=m  TranslationZOffset=0  TranslationZOffsetUnits=m  TranslationThetaOffset=0  TranslationThetaOffsetUnits=deg  RotationMethod=None  RotationAngleUnits=deg  RotationStandardAxis=+Z  RotationAngle=90  RotationArbitraryAxis=[1 0 0]  FollAlignAxisA=+X  BaseAlignAxisA=+Y  FollAlignAxisB=+Y  BaseAlignAxisB=+Z  RotationSequenceAxes=FollowerAxes  RotationSequence=XYX  RotationSequenceAngles=[0 0 0]  RotationSequenceAnglesUnits=deg  RotationMatrix=[1 0 0; 0 1 0; 0 0 1]
  Cable : Subsystem
  Conn_Plate : sm_lib/Body Elements/Brick Solid  GraphicAmbientColor=[0.15 0.15 0.15 1.0]  BasedOnType=Mass  BrickDimensions=[L.ap*2 P.d P.h]  BrickDimensionUnits=mm  CenterOfMass=[0 0 0]  CenterOfMassUnits=m  GraphicDiffuseColor=[0.0 0.2 1.0]  Density=0  DensityUnits=g/cm^3  DoExposeReferenceFrame=on  GraphicEmissiveColor=[0.0 0.0 0.0 1.0]  ExportEntireGeometry=off  SerializedFrames=<Frames/>  MarkerShape=Sphere  MarkerSize=10  GraphicType=FromGeometry  InertiaType=CalculateFromGeometry  Mass=L.cpmass  MassUnits=kg  MomentsOfInertia=[1 1 1]  MomentsOfInertiaUnits=kg*m^2  GraphicOpacity=1.0  ProductsOfInertia=[0 0 0]  ProductsOfInertiaUnits=kg*m^2  GraphicShininess=75  GraphicSpecularColor=[0.5 0.5 0.5 1.0]  GraphicVisPropType=SimpleVisualProperties
  Load init position2 : sm_lib/Frames and Transforms/Rigid Transform  TranslationMethod=Cartesian  TranslationStandardOffset=0  TranslationLengthUnit=mm  TranslationStandardAxis=+Z  TranslationCartesianOffset=[0 -L.height*.5-P.d 0 ]  TranslationROffset=0  TranslationROffsetUnits=m  TranslationZOffset=0  TranslationZOffsetUnits=m  TranslationThetaOffset=0  TranslationThetaOffsetUnits=deg  RotationMethod=None  RotationAngleUnits=deg  RotationStandardAxis=+X  RotationAngle=180  RotationArbitraryAxis=[0 0 1]  FollAlignAxisA=+X  BaseAlignAxisA=+Y  FollAlignAxisB=+Y  BaseAlignAxisB=+Z  RotationSequenceAxes=FollowerAxes  RotationSequence=XYX  RotationSequenceAngles=[0 0 0]  RotationSequenceAnglesUnits=deg  RotationMatrix=[1 0 0; 0 1 0; 0 0 1]
  Load init position3 : sm_lib/Frames and Transforms/Rigid Transform  TranslationMethod=Cartesian  TranslationStandardOffset=0  TranslationLengthUnit=mm  TranslationStandardAxis=+Z  TranslationCartesianOffset=[0 -P.d*0.5-L.height*0.5 -P.h*.5 ]  TranslationROffset=0  TranslationROffsetUnits=m  TranslationZOffset=0  TranslationZOffsetUnits=m  TranslationThetaOffset=0  TranslationThetaOffsetUnits=deg  RotationMethod=StandardAxis  RotationAngleUnits=deg  RotationStandardAxis=+Y  RotationAngle=180  RotationArbitraryAxis=[0 0 1]  FollAlignAxisA=+X  BaseAlignAxisA=+Y  FollAlignAxisB=+Y  BaseAlignAxisB=+Z  RotationSequenceAxes=FollowerAxes  RotationSequence=XYX  RotationSequenceAngles=[0 0 0]  RotationSequenceAnglesUnits=deg  RotationMatrix=[1 0 0; 0 1 0; 0 0 1]
  Load1 : sm_lib/Body Elements/Brick Solid  GraphicAmbientColor=[0.15 0.15 0.15 1.0]  BasedOnType=Mass  BrickDimensions="[L.width*2 L.height  L.depth]"  BrickDimensionUnits=mm  CenterOfMass=[0 0 0]  CenterOfMassUnits=m  GraphicDiffuseColor=[0.6 0.6 1.0]  Density=L.den  DensityUnits=g/cm^3  DoExposeReferenceFrame=off  GraphicEmissiveColor=[0.0 0.0 0.0 1.0]  ExportEntireGeometry=off  SerializedFrames=<Frames><Frame><Id>Frame1</Id><Value><Name>F</Name><Origin><Source>ReferenceFrame</Source><FeatureName></FeatureName></Origin><PrimaryAxis><DefinedDirection>+Z</DefinedDirection><Source>ReferenceFrame</Source><SourceDirection>+Z</SourceDirection><FeatureName></FeatureName></PrimaryAxis><SecondaryAxis><DefinedDirection>+X</DefinedDirection><Source>ReferenceFrame</Source><SourceDirection>+X</SourceDirection><FeatureName></FeatureName></SecondaryAxis></Value></Frame></Frames>  MarkerShape=Sphere  MarkerSize=10  GraphicType=FromGeometry  InertiaType=CalculateFromGeometry  Mass=L.mass*2  MassUnits=kg  MomentsOfInertia=[0 0 0]  MomentsOfInertiaUnits=kg*m^2  GraphicOpacity=1.0  ProductsOfInertia=[0 0 0]  ProductsOfInertiaUnits=kg*m^2  GraphicShininess=75  GraphicSpecularColor=[0.5 0.5 0.5 1.0]  GraphicVisPropType=SimpleVisualProperties
  Load1 Rotation1 : sm_lib/Frames and Transforms/Rigid Transform  TranslationMethod=None  TranslationStandardOffset=0  TranslationLengthUnit=m  TranslationStandardAxis=+Z  TranslationCartesianOffset=[0 0 0]  TranslationROffset=0  TranslationROffsetUnits=m  TranslationZOffset=0  TranslationZOffsetUnits=m  TranslationThetaOffset=0  TranslationThetaOffsetUnits=deg  RotationMethod=StandardAxis  RotationAngleUnits=deg  RotationStandardAxis=+X  RotationAngle=90  RotationArbitraryAxis=[0 0 1]  FollAlignAxisA=+Y  BaseAlignAxisA=-Z  FollAlignAxisB=+X  BaseAlignAxisB=+X  RotationSequenceAxes=FollowerAxes  RotationSequence=XYX  RotationSequenceAngles=[0 0 0]  RotationSequenceAnglesUnits=deg  RotationMatrix=[1 0 0; 0 1 0; 0 0 1]
  Planar Load1 : Subsystem
  Rigid Transform24 : sm_lib/Frames and Transforms/Rigid Transform  TranslationMethod=Cartesian  TranslationStandardOffset=0  TranslationLengthUnit=mm  TranslationStandardAxis=+Z  TranslationCartesianOffset=[-0.5*(P.d+P.Bd) 0.5*T.rs 0]  TranslationROffset=0  TranslationROffsetUnits=m  TranslationZOffset=0  TranslationZOffsetUnits=m  TranslationThetaOffset=0  TranslationThetaOffsetUnits=deg  RotationMethod=StandardAxis  RotationAngleUnits=deg  RotationStandardAxis=+Y  RotationAngle=180  RotationArbitraryAxis=[1 0 0]  FollAlignAxisA=+X  BaseAlignAxisA=+Y  FollAlignAxisB=+Y  BaseAlignAxisB=+Z  RotationSequenceAxes=FollowerAxes  RotationSequence=XYX  RotationSequenceAngles=[0 0 0]  RotationSequenceAnglesUnits=deg  RotationMatrix=[1 0 0; 0 1 0; 0 0 1]
  Rigid Transform26 : sm_lib/Frames and Transforms/Rigid Transform  TranslationMethod=Cartesian  TranslationStandardOffset=0  TranslationLengthUnit=mm  TranslationStandardAxis=+Z  TranslationCartesianOffset=[0.5*(P.d+P.Bd) 0.5*T.rs 0]  TranslationROffset=0  TranslationROffsetUnits=m  TranslationZOffset=0  TranslationZOffsetUnits=m  TranslationThetaOffset=0  TranslationThetaOffsetUnits=deg  RotationMethod=StandardAxis  RotationAngleUnits=deg  RotationStandardAxis=+Y  RotationAngle=180  RotationArbitraryAxis=[1 0 0]  FollAlignAxisA=+X  BaseAlignAxisA=+Y  FollAlignAxisB=+Y  BaseAlignAxisB=+Z  RotationSequenceAxes=FollowerAxes  RotationSequence=XYX  RotationSequenceAngles=[0 0 0]  RotationSequenceAnglesUnits=deg  RotationMatrix=[1 0 0; 0 1 0; 0 0 1]
  graph1 : sm_lib/Body Elements/Extruded Solid  GraphicAmbientColor=[0.15 0.15 0.15 1.0]  BasedOnType=Density  CenterOfMass=[0 0 0]  CenterOfMassUnits=m  GraphicDiffuseColor=[0.6 0.6 0.0]  ExportConvexHullGeometry=off  ExtrusionCrossSection=0.5*P.d*[3,0; 3,1; 3/2,2; -3/2,2; -3,1; -3,0]  ExtrusionCrossSectionUnits=mm  Density=0  DensityUnits=g/cm^3  DoExposeReferenceFrame=on  GraphicEmissiveColor=[0.0 0.0 0.0 1.0]  ExportEntireGeometry=off  ExtrusionLength=P.h  ExtrusionLengthUnits=mm  ExtrusionType=General  SerializedFrames=<Frames/>  MarkerShape=Sphere  MarkerSize=10  GraphicType=FromGeometry  InertiaType=CalculateFromGeometry  Mass=0  MassUnits=kg  MomentsOfInertia=[1 1 1]  MomentsOfInertiaUnits=kg*m^2  PolygonNumSides=6  GraphicOpacity=1.0  PolygonOuterRadius=1  PolygonOuterRadiusUnits=m  ProductsOfInertia=[0 0 0]  ProductsOfInertiaUnits=kg*m^2  GraphicShininess=75  GraphicSpecularColor=[0.5 0.5 0.5 1.0]  GraphicVisPropType=SimpleVisualProperties
  graph2 : sm_lib/Body Elements/Extruded Solid  GraphicAmbientColor=[0.15 0.15 0.15 1.0]  BasedOnType=Density  CenterOfMass=[0 0 0]  CenterOfMassUnits=m  GraphicDiffuseColor=[0.6 0.6 0.0]  ExportConvexHullGeometry=off  ExtrusionCrossSection=0.5*P.d*[3,0; 3,1; 3/2,2; -3/2,2; -3,1; -3,0]  ExtrusionCrossSectionUnits=mm  Density=0  DensityUnits=g/cm^3  DoExposeReferenceFrame=on  GraphicEmissiveColor=[0.0 0.0 0.0 1.0]  ExportEntireGeometry=off  ExtrusionLength=P.h  ExtrusionLengthUnits=mm  ExtrusionType=General  SerializedFrames=<Frames/>  MarkerShape=Sphere  MarkerSize=10  GraphicType=FromGeometry  InertiaType=CalculateFromGeometry  Mass=0  MassUnits=kg  MomentsOfInertia=[1 1 1]  MomentsOfInertiaUnits=kg*m^2  PolygonNumSides=6  GraphicOpacity=c.opac  PolygonOuterRadius=1  PolygonOuterRadiusUnits=m  ProductsOfInertia=[0 0 0]  ProductsOfInertiaUnits=kg*m^2  GraphicShininess=75  GraphicSpecularColor=[0.5 0.5 0.5 1.0]  GraphicVisPropType=SimpleVisualProperties
  graph3 : sm_lib/Body Elements/Brick Solid  GraphicAmbientColor=[0.15 0.15 0.15 1.0]  BasedOnType=Density  BrickDimensions=[P.d P.h P.d*.5]  BrickDimensionUnits=mm  CenterOfMass=[0 0 0]  CenterOfMassUnits=m  GraphicDiffuseColor=[0.6 0.6 0.0]  Density=0  DensityUnits=g/cm^3  DoExposeReferenceFrame=on  GraphicEmissiveColor=[0.0 0.0 0.0 1.0]  ExportEntireGeometry=off  SerializedFrames=<Frames/>  MarkerShape=Sphere  MarkerSize=10  GraphicType=FromGeometry  InertiaType=CalculateFromGeometry  Mass=0  MassUnits=kg  MomentsOfInertia=[1 1 1]  MomentsOfInertiaUnits=kg*m^2  GraphicOpacity=1.0  ProductsOfInertia=[0 0 0]  ProductsOfInertiaUnits=kg*m^2  GraphicShininess=75  GraphicSpecularColor=[0.5 0.5 0.5 1.0]  GraphicVisPropType=SimpleVisualProperties
  graph4 : sm_lib/Body Elements/Brick Solid  GraphicAmbientColor=[0.15 0.15 0.15 1.0]  BasedOnType=Density  BrickDimensions=[P.d P.h P.d*.5]  BrickDimensionUnits=mm  CenterOfMass=[0 0 0]  CenterOfMassUnits=m  GraphicDiffuseColor=[0.6 0.6 0.0]  Density=0  DensityUnits=g/cm^3  DoExposeReferenceFrame=on  GraphicEmissiveColor=[0.0 0.0 0.0 1.0]  ExportEntireGeometry=off  SerializedFrames=<Frames/>  MarkerShape=Sphere  MarkerSize=10  GraphicType=FromGeometry  InertiaType=CalculateFromGeometry  Mass=0  MassUnits=kg  MomentsOfInertia=[1 1 1]  MomentsOfInertiaUnits=kg*m^2  GraphicOpacity=1.0  ProductsOfInertia=[0 0 0]  ProductsOfInertiaUnits=kg*m^2  GraphicShininess=75  GraphicSpecularColor=[0.5 0.5 0.5 1.0]  GraphicVisPropType=SimpleVisualProperties
  Conn1 : PMIOPort  Side=Left
  Pulley low 1 : PMIOPort  Port=2  Side=Right
  Pullley low 2 : PMIOPort  Port=3  Side=Right
  LoadFrame : PMIOPort  Port=4  Side=Left
  wires:
  cable mass/1 -> Cable/1(In1)
  connections:
  Conn_Plate/RConn1 -- Load init position3/LConn1 -- " 17"/RConn1
  Rigid Transform24/LConn1 -- Rigid Transform26/LConn1 -- " "/LConn1 -- " 17"/LConn1 -- " 4"/LConn1 -- " 5"/LConn1 -- Cable/RConn1 -- Load init position2/RConn1 -- " 3"/LConn1
  Load init position3/RConn1 -- Load1/LConn1 -- LoadFrame/RConn1
  Load1 Rotation1/LConn1 -- Planar Load1/RConn1
  graph4/RConn1 -- " "/RConn1
  graph1/RConn1 -- " 3"/RConn1
  " 4"/RConn1 -- graph3/RConn1
  " 5"/RConn1 -- graph2/RConn1
  Load init position2/LConn1 -- Load1 Rotation1/RConn1
  Planar Load1/LConn1 -- Conn1/RConn1
  Pulley low 1/RConn1 -- Rigid Transform24/RConn1
  Pullley low 2/RConn1 -- Rigid Transform26/RConn1

== system DemonstratorSimscape/Transmission System/Anchor and Load/Sheave_03/Bending loss ==
  Sin (kN) : Inport
  w (deg/s) : Inport  Port=2
  Add : Sum
  Add1 : Sum  Inputs=+-
  Constant : Constant
  Constant2 : Constant
  Math Function : Math  Operator=pow  SignedPower=on  SaturateOnIntegerOverflow=on
  Product : Product
  Product1 : Product
  Scope : Scope
  dT_Gain : Gain  Gain=0
  dr for positive omega : Constant
  dr switch : MATLAB Function  TreatAsAtomicUnit=on
  eta_sh : Constant  Value=eta_sh
  torque (Nm) : Gain  Gain=r_sheave
  dT (Nm) : Outport  VectorParamsAs1DForOutWhenUnconnected=off
  Sout (kN) : Outport  Port=2  VectorParamsAs1DForOutWhenUnconnected=off
  wires:
  Add/1 -> Math Function/1
  Sin (kN)/1 -> Product1/2, Product/2
  torque (Nm)/1 -> Scope/1, dT_Gain/1
  Math Function/1 -> Add1/1, Product1/1
  Add1/1 -> Product/1
  Product/1 -> torque (Nm)/1
  eta_sh/1 -> Add/2
  Constant/1 -> Add/1
  Constant2/1 -> Add1/2
  Product1/1 -> Sout (kN)/1
  dT_Gain/1 -> dT (Nm)/1
  dr for positive omega/1 -> dr switch/2(dr_wpos)
  dr switch/1(dr) -> Math Function/2
  w (deg/s)/1 -> dr switch/1(w)

== system DemonstratorSimscape/Transmission System/Anchor and Load/Sheave_03/PS>Sim1 ==
  b (deg/s^2) : nesl_utility/PS-Simulink Converter  PhysicalDomain=network_engine_domain  SubClassName=ps_output  LeftPortType=input  RightPortType=output  PseudoPeriodic=off  Frequencies=[]  Unit=deg/s^2  AffineConversion=off
  fc (N) : nesl_utility/PS-Simulink Converter  PhysicalDomain=network_engine_domain  SubClassName=ps_output  LeftPortType=input  RightPortType=output  PseudoPeriodic=off  Frequencies=[]  Unit=N  AffineConversion=off
  ft (N) : nesl_utility/PS-Simulink Converter  PhysicalDomain=network_engine_domain  SubClassName=ps_output  LeftPortType=input  RightPortType=output  PseudoPeriodic=off  Frequencies=[]  Unit=N  AffineConversion=off
  q (deg) : nesl_utility/PS-Simulink Converter  PhysicalDomain=network_engine_domain  SubClassName=ps_output  LeftPortType=input  RightPortType=output  PseudoPeriodic=off  Frequencies=[]  Unit=deg  AffineConversion=off
  t (Nm) : nesl_utility/PS-Simulink Converter  PhysicalDomain=network_engine_domain  SubClassName=ps_output  LeftPortType=input  RightPortType=output  PseudoPeriodic=off  Frequencies=[]  Unit=N*m  AffineConversion=off
  tc (Nm) : nesl_utility/PS-Simulink Converter  PhysicalDomain=network_engine_domain  SubClassName=ps_output  LeftPortType=input  RightPortType=output  PseudoPeriodic=off  Frequencies=[]  Unit=N*m  AffineConversion=off
  tt (Nm) : nesl_utility/PS-Simulink Converter  PhysicalDomain=network_engine_domain  SubClassName=ps_output  LeftPortType=input  RightPortType=output  PseudoPeriodic=off  Frequencies=[]  Unit=N*m  AffineConversion=off
  w (deg/s) : nesl_utility/PS-Simulink Converter  PhysicalDomain=network_engine_domain  SubClassName=ps_output  LeftPortType=input  RightPortType=output  PseudoPeriodic=off  Frequencies=[]  Unit=deg/s  AffineConversion=off
  q : PMIOPort  Side=Left
  Conn2 : PMIOPort  Port=2  Side=Left
  Conn3 : PMIOPort  Port=3  Side=Left
  Conn4 : PMIOPort  Port=4  Side=Left
  Conn5 : PMIOPort  Port=5  Side=Left
  Conn6 : PMIOPort  Port=6  Side=Left
  Conn7 : PMIOPort  Port=7  Side=Left
  Conn8 : PMIOPort  Port=8  Side=Left
  Out1 : Outport  VectorParamsAs1DForOutWhenUnconnected=off
  Out2 : Outport  Port=2  VectorParamsAs1DForOutWhenUnconnected=off
  Out3 : Outport  Port=3  VectorParamsAs1DForOutWhenUnconnected=off
  Out4 : Outport  Port=4  VectorParamsAs1DForOutWhenUnconnected=off
  Out5 : Outport  Port=5  VectorParamsAs1DForOutWhenUnconnected=off
  Out6 : Outport  Port=6  VectorParamsAs1DForOutWhenUnconnected=off
  Out7 : Outport  Port=7  VectorParamsAs1DForOutWhenUnconnected=off
  Out8 : Outport  Port=8  VectorParamsAs1DForOutWhenUnconnected=off
  wires:
  tt (Nm)/1 -> Out8/1
  ft (N)/1 -> Out7/1
  tc (Nm)/1 -> Out6/1
  fc (N)/1 -> Out5/1
  t (Nm)/1 -> Out4/1
  b (deg/s^2)/1 -> Out3/1
  w (deg/s)/1 -> Out2/1
  q (deg)/1 -> Out1/1
  connections:
  Conn8/RConn1 -- tt (Nm)/LConn1
  ft (N)/LConn1 -- Conn7/RConn1
  Conn6/RConn1 -- tc (Nm)/LConn1
  fc (N)/LConn1 -- Conn5/RConn1
  Conn4/RConn1 -- t (Nm)/LConn1
  Conn3/RConn1 -- b (deg/s^2)/LConn1
  Conn2/RConn1 -- w (deg/s)/LConn1
  q/RConn1 -- q (deg)/LConn1
